simulink model "dev_WaterSide"  (R2020b)
settings: Solver=VariableStepAuto  StartTime=0.0  StopTime=800  RelTol=1e-3
libraries: simulink x2, powerlib_meascontrol x1, simulink_extras x1, IMT_Library x1
settings Model: Creator=Mr_Li  LastModifiedBy=Mr_Li
settings SolverCC: ZeroCrossAlgorithm=Adaptive
settings DebuggingCC: IgnoredZcDiagnostic=none

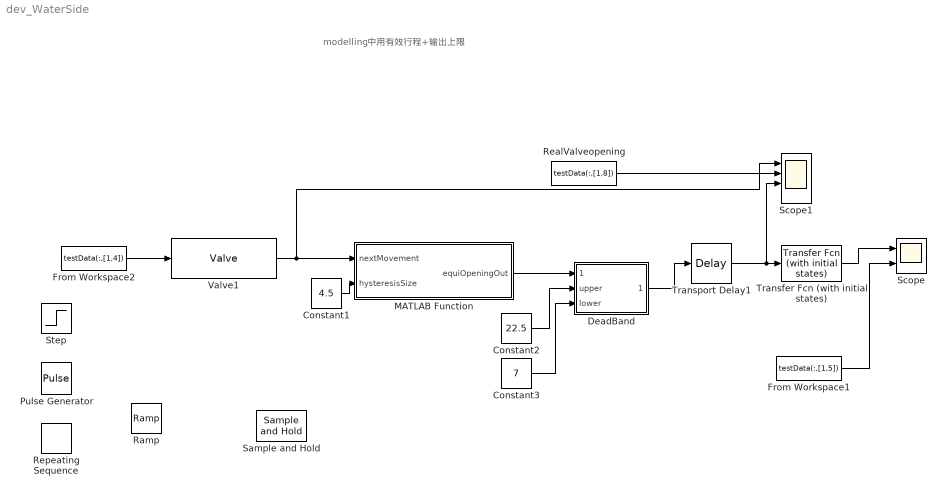
== system dev_WaterSide ==
  note: modelling中用有效行程+输出上限
  Constant1 : Constant  Value=4.5
  Constant2 : Constant  Value=22.5
  Constant3 : Constant  Value=7
  DeadBand : MATLAB Function  TreatAsAtomicUnit=on
  From Workspace1 : FromWorkspace  VariableName=testData(:,[1,5])
  From Workspace2 : FromWorkspace  VariableName=testData(:,[1,4])  SampleTime=1
  MATLAB Function : MATLAB Function  TreatAsAtomicUnit=on
  Pulse Generator : DiscretePulseGenerator  PulseType=Time based  Amplitude=100  Period=500  PulseWidth=50  PhaseDelay=50
  Ramp : simulink/Sources/Ramp  slope=1  start=0  InitialOutput=0
  RealValveopening : FromWorkspace  VariableName=testData(:,[1,8])
  Repeating Sequence : simulink/Sources/Repeating Sequence  rep_seq_t=[0 60 120]  rep_seq_y=[0 10 0 ]
  Sample and Hold : powerlib_meascontrol/Additional Components/Sample and Hold  ic=0  Ts=0
      settings: SourceProductBaseCode=PS
  Scope : Scope  NumInputPorts=2
  Scope1 : Scope  NumInputPorts=4
  Step : Step  Time=10  After=100  SampleTime=0
  Transfer Fcn (with initial states) : simulink_extras/Additional Linear/Transfer Fcn (with initial states)  N=[0.032]  D=[3.6 1]  X0=0
  Transport Delay1 : TransportDelay  DelayTime=3
  Valve1 : IMT_Library/Valve  upper=101  lower=1.2  movementThreshold=1
      settings: SourceProductName=Imitation
  wires:
  Transfer Fcn (with initial states)/1 -> Scope/1
  Constant1/1 -> MATLAB Function/2(hysteresisSize)
  Constant2/1 -> DeadBand/2(upper)
  Constant3/1 -> DeadBand/3(lower)
  DeadBand/1(realOut) -> Transport Delay1/1
  From Workspace1/1 -> Scope/2
  MATLAB Function/1(equiOpeningOut) -> DeadBand/1(current)
  RealValveopening/1 -> Scope1/2
  Valve1/1 -> MATLAB Function/1(nextMovement), Scope1/1
  Transport Delay1/1 -> Scope1/3, Transfer Fcn (with initial states)/1
  From Workspace2/1 -> Valve1/1

== matlab function dev_WaterSide/MATLAB Function ==
  settings: updateMethod=DISCRETE
  data: nextMovement input; equiOpeningOut output; hysteresisSize input
function equiOpeningOut  = fcn(nextMovement,hysteresisSize)
%[equiOpeningOut,previousDirectionOut]
persistent previousDirection; %阀门移动是否同向,默认true为上升
persistent hysteresisBuffer;
persistent equiOpening; %阀门等效开度，带缓存
persistent currentValve; %缓存上一步的阀门开度，实际的阀门开度

% 静态变量初始化
if(isempty(currentValve))
    currentValve=nextMovement;
end

if(isempty(equiOpening))
    equiOpening=nextMovement;
end

if(isempty(previousDirection))
    previousDirection=true;
%     previousDirectionOut=previousDirection;
    hysteresisBuffer=hysteresisSize;
end

if(nextMovement==currentValve)
    equiOpeningOut=equiOpening;
%     previousDirectionOut=previousDirection;
    return;
end

% 判断阀门运动方向
if(((nextMovement-currentValve)>=0)~=previousDirection)
    if(abs(currentValve-nextMovement)>0.1)
        %避免等效下降速度快于实际，而产生的方向误改变情况
        previousDirection=((nextMovement-currentValve)>=0);%equiOpening
%         previousDirectionOut=previousDirection;
        hysteresisBuffer=hysteresisSize;
    end
%     previousDirectionOut=previousDirection;
end

% 计算实际阀门增量和buffer
hysteresisBuffer=hysteresisBuffer-abs(currentValve-nextMovement);


% 计算buffer后的
if(hysteresisBuffer<=0)
%     表明抵消完buffer或者抵消完buffer后还有多余增量
    if(previousDirection)% 为什么没有三目表达式
        equiOpening=equiOpening+abs(hysteresisBuffer);
        equiOpeningOut=equiOpening;
        currentValve=nextMovement;
    else
        equiOpening=equiOpening+abs(hysteresisBuffer)*(-1);
        equiOpeningOut=equiOpening;
        currentValve=nextMovement;
    end
%     previousDirectionOut=previousDirection;
    hysteresisBuffer=0;
else
%     equiOpening=currentValve;
    equiOpeningOut=equiOpening;
    currentValve=nextMovement;
%     previousDirectionOut=previousDirection;
end

== matlab function dev_WaterSide/DeadBand ==
  settings: updateMethod=CONTINUOUS
  data: current input; upper input; realOut output; lower input
function realOut = deadBandLimit(current,upper,lower)
if(current<=lower)
    realOut = 0;
elseif(current>upper)
    realOut=upper;
else
    realOut=current;
end
